simulink model "PlutoSpectrumSave"  (R2023a)
settings: Solver=VariableStepAuto  StartTime=0.0  StopTime=10.0  RelTol=1e-3
values from neighbouring files (symbols this model uses):
  Fs = 1e6    (= 1000000)    [generateWave.m]    (also in rfDataProcessing.m)
undefined symbols (not defined in the file or in its folder): ip, usb
libraries: plutoradiolib x1
settings Model: Creator=joonheelee  LastModifiedBy=joonheelee

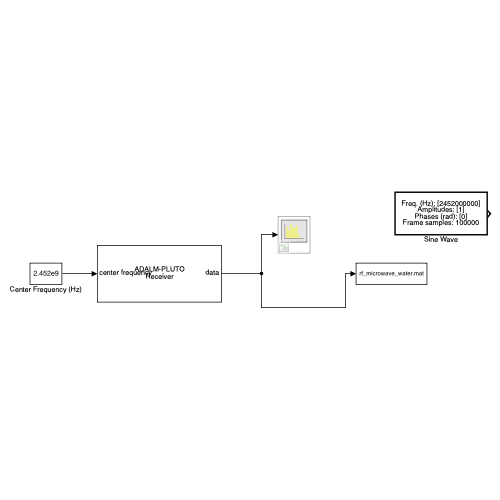
[thumbnail: Simulink's stored preview of the top-level diagram]
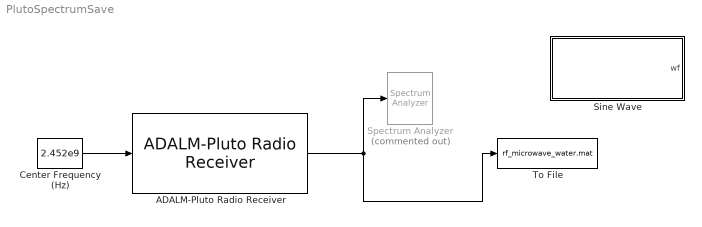
== system PlutoSpectrumSave ==
  ADALM-Pluto Radio Receiver : plutoradiolib/ADALM-Pluto Radio Receiver  RadioID=usb:0  uri=ip:10.0.0.200  CenterFrequencySource=Input Port  CenterFrequency=2.4e9  GainSource=AGC Slow Attack  GainSourceBlock=AGC Slow Attack  Gain=50  ChannelMapping=1  BasebandSampleRate=2e6  OutputDataType=double  SamplesPerFrame=2000  OverflowOutputPort=off  EnableBurstMode=off  NumFramesInBurst=1  ShowAdvancedProperties=off  UseCustomFilter=off  filtPathRates=[737280000 11520000 3840000 1920000 960000 240000]  filtCoefficients=[-192 82 85 -215 228 -102 -110 290 -318 145 160 -426 471 -215 -238 633 -697 318 349 -923 1009 -457 -498 1309 -1423 640 693 -1812 1959 -876 -945 2458 -2647 1180 1268 -3290 3534 -1572 -1688 4375 -4698 2091 2247 -5836 6284 -2807 -3031 7918 -8588 3870 4225 -11182 12324 -5662 -6330 17255 -19735 9507 11312 -33568 43355 -25227 -42139 305542 305542 -42139 -25227 43355 -33568 11312 9507 -19735 17255 -6330 -5662 12324 -11182 4225 3870 -8588 7918 -3031 -2807 6284 -5836 2247 2091 -4698 4375 -1688 -1572 3534 -3290 1268 1180 -2647 2458 -945 -876 1959 -1812 693 640 -1423 1309 -498 -457 1009 -923 349 318 -697 633 -238 -215 471 -426 160 145 -318 290 -110 -102 228 -215 85 82 -192]  filtCoefficientSize=128  filtDecimInterpFactor=4  filtGain=-12  filtRFBandwidth=18000000  filterConfigStruct=struct()  EnableQuadratureCorrection=on  EnableRFDCCorrection=on  EnableBasebandDCCorrection=on  FrequencyCorrection=0  OverrideSampleTime=off  SampleTime=0.02  DataTimeout=Inf  ENSMPinControlMode=None  BISTLoopbackMode=Disabled  BISTToneInject=Disabled  BISTSignalGen=PRBS  BISTToneFreq=Fs/32  BISTToneLevel=0
  Center Frequency (Hz) : Constant  Value=2.452e9
  Sine Wave : MATLAB Function  Tag=BlockGeneratedWWGApp  TreatAsAtomicUnit=on  SystemSampleTime=0.0010000000000000000208  mask(Sine Wave Generator){nsamps=1, OutputAfterFinalValue=Cyclic repetition}
      mask prompts: nsamps "Samples per frame:"; OutputAfterFinalValue "Form output after final data value by:"
      mask init:
      | %% Generating Sine Wave waveform
      | Fs = 1000; 								 % Specify the sample rate of the waveform in Hz
      | 
      | % Sine Wave configuration
      | % waveform configuration:
      | sineWaves = dsp.SineWave('Frequency', 2452000000, ...
      |     'Amplitude', 1, ...
      |     'PhaseOffset', 0, ...
      |     'SampleRate', Fs , ...
      |     'ComplexOutput', 0, ...
      |     'SamplesPerFrame', 100 *Fs);
      | 
      | % Generation
      | waveform = sineWaves();
      | 
      | %% Configuring block: update parameters and UserData
      | % Get current block
      | thisBlock = gcb;
      | 
      | % Set info parameters
      | maskHandle = Simulink.Mask.get(thisBlock);
      | textFsDialog = maskHandle.getDialogControl('textFs');
      | textFsDialog.Prompt = ['Waveform sample rate (Fs): ' num2str(Fs*1e-6,'%.9g') ' MHz'];
      | textWfLengthDialog = maskHandle.getDialogControl('textWFLength');
      | textWfLengthDialog.Prompt = ['Waveform length: ' num2str(length(waveform)) ' samples'];
      | 
      | % Set sample time of the block
      | set_param(thisBlock, 'SystemSampleTime', num2str(nsamps/Fs,'%.20g'));
      | 
      | % Update UserData
      | outVar.WaveformConfig = sineWaves;
      | outVar.WaveformLength = length(waveform);
      | outVar.Fs = Fs;
      | set_param(thisBlock, 'UserData', outVar);
  Spectrum Analyzer : SpectrumAnalyzer  Commented=on  WindowPosition=[496.000000,310.000000,800.000000,500.000000,]  ScopeFrameLocation=window  YLimits=[-0.8689639,39.78345711]  ColorLimits=[-80 20]  SelectedToolstripTab=spectrumAnalyzerToolstrip.estimationTab
  To File : ToFile  Filename=rf_microwave_water.mat  MatrixName=data  SaveFormat=Timeseries
  wires:
  ADALM-Pluto Radio Receiver/1 -> To File/1, Spectrum Analyzer/1
  Center Frequency (Hz)/1 -> ADALM-Pluto Radio Receiver/1

== matlab function PlutoSpectrumSave/Sine Wave ==
  data: wf output; waveform parameter; nsamps parameter; OutputAfterFinalValue parameter
function wf = wfGenerator(waveform, nsamps, OutputAfterFinalValue)

% Create persistent variable
persistent src;

% Preallocate output
wf = complex(zeros(nsamps,size(waveform,2)));

if isempty(src)
    % Get action when signal ends
    if OutputAfterFinalValue == 1
        signalEndAction = 'Cyclic repetition';
    else
        signalEndAction = 'Set to zero';
    end
    
    % Initialize persistent dsp.SignalSource to get current frame
    src = dsp.SignalSource(waveform,nsamps,'SignalEndAction',signalEndAction);
end

% Extract current frame
wf(:,:) = src();

end
